simulink model "rocket_state_sim_2020b"  (R2020b)
settings: Solver=VariableStepAuto  StartTime=0.0  StopTime=t_sim  MaxStep=1e-3  RelTol=1e-5  AbsTol=1e-3
undefined symbols (not defined in the file): M, r0, v0
libraries: SKYWARD_LIB x3
settings Model: Creator=alem1  LastModifiedBy=aless
settings SolverCC: AutoScaleAbsTol=off

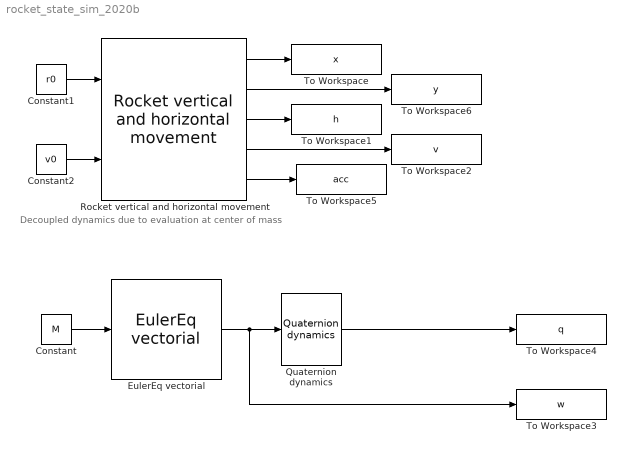
== system rocket_state_sim_2020b ==
  note: Decoupled dynamics due to evaluation at center of mass
  Constant : Constant  Value=M
  Constant1 : Constant  Value=r0
  Constant2 : Constant  Value=v0
  EulerEq vectorial : SKYWARD_LIB/EulerEq vectorial  SystemSampleTime=-1  VariantActivationTime=update diagram  Latency=0  AutoFrameSizeCalculation=off
  Quaternion dynamics : SKYWARD_LIB/Quaternion dynamics  SystemSampleTime=-1  VariantActivationTime=update diagram  Latency=0  AutoFrameSizeCalculation=off
  Rocket vertical and horizontal movement : SKYWARD_LIB/Rocket vertical and horizontal movement  SystemSampleTime=-1  VariantActivationTime=update diagram  Latency=0  AutoFrameSizeCalculation=off
  To Workspace : ToWorkspace  VariableName=x  SampleTime=-1
  To Workspace1 : ToWorkspace  VariableName=h  SampleTime=-1
  To Workspace2 : ToWorkspace  VariableName=v  SampleTime=-1
  To Workspace3 : ToWorkspace  VariableName=w  SampleTime=-1
  To Workspace4 : ToWorkspace  VariableName=q  SampleTime=-1
  To Workspace5 : ToWorkspace  VariableName=acc  SampleTime=-1
  To Workspace6 : ToWorkspace  VariableName=y  SampleTime=-1
  wires:
  Constant1/1 -> Rocket vertical and horizontal movement/1
  Constant2/1 -> Rocket vertical and horizontal movement/2
  Rocket vertical and horizontal movement/1 -> To Workspace/1
  EulerEq vectorial/1 -> To Workspace3/1, Quaternion dynamics/1
  Constant/1 -> EulerEq vectorial/1
  Quaternion dynamics/1 -> To Workspace4/1
  Rocket vertical and horizontal movement/3 -> To Workspace1/1
  Rocket vertical and horizontal movement/4 -> To Workspace2/1
  Rocket vertical and horizontal movement/5 -> To Workspace5/1
  Rocket vertical and horizontal movement/2 -> To Workspace6/1
